simulink model "SIL_OlfatiSaber"  (R2021b)
settings: Solver=FixedStepDiscrete  StartTime=0  StopTime=T  FixedStep=0.01  RelTol=1e-3  EnableMultiTasking=on
model workspace (MAT data in the model file):
  SL_ROS_VariableLengthArrays_MaxSizes : object (value not decoded)
values from neighbouring files (symbols this model uses):
  airspeed_ref = 42    [start_swarm.m]
  altitude_ref = 300    [start_swarm.m]
  N_Waypoints = size(Waypoints,1)    [start_swarm.m]
  radius_waypoint = 200    [start_swarm.m]
  Waypoints = [1200 -1000 ... (first row only)    [start_swarm.m]
undefined symbols (not defined in the file or in its folder): DiscIntNeverNeededParam, Elevators, p_swarm, Propeller, RightAileron, RightFlap, Rudder
libraries: robotlib x36, slpidlib x15, eeGeneralControl x5, simulink x5
(part 4 of 5)

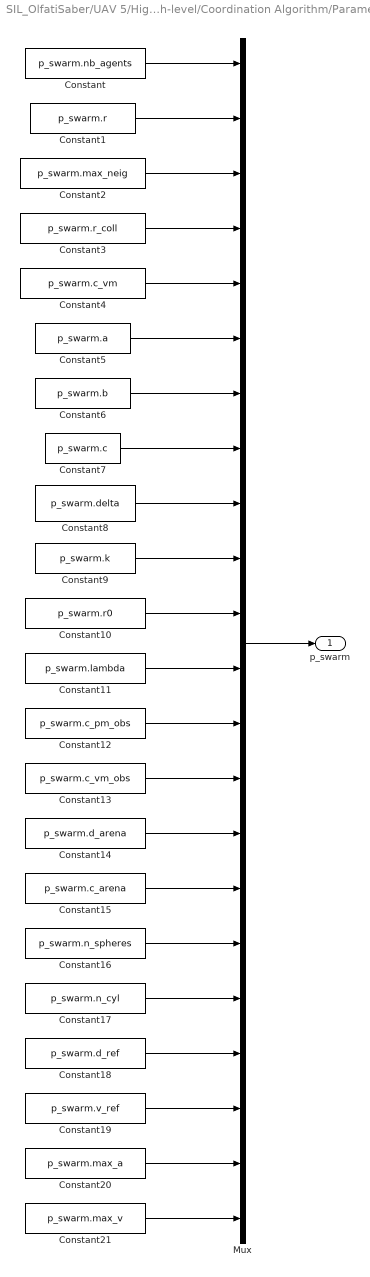
== system SIL_OlfatiSaber/UAV 5/High-level/Coordination Algorithm/Parameters ==
  Constant : Constant  Value=p_swarm.nb_agents
  Constant1 : Constant  Value=p_swarm.r
  Constant10 : Constant  Value=p_swarm.r0
  Constant11 : Constant  Value=p_swarm.lambda
  Constant12 : Constant  Value=p_swarm.c_pm_obs
  Constant13 : Constant  Value=p_swarm.c_vm_obs
  Constant14 : Constant  Value=p_swarm.d_arena
  Constant15 : Constant  Value=p_swarm.c_arena
  Constant16 : Constant  Value=p_swarm.n_spheres
  Constant17 : Constant  Value=p_swarm.n_cyl
  Constant18 : Constant  Value=p_swarm.d_ref
  Constant19 : Constant  Value=p_swarm.v_ref
  Constant2 : Constant  Value=p_swarm.max_neig
  Constant20 : Constant  Value=p_swarm.max_a
  Constant21 : Constant  Value=p_swarm.max_v
  Constant3 : Constant  Value=p_swarm.r_coll
  Constant4 : Constant  Value=p_swarm.c_vm
  Constant5 : Constant  Value=p_swarm.a
  Constant6 : Constant  Value=p_swarm.b
  Constant7 : Constant  Value=p_swarm.c
  Constant8 : Constant  Value=p_swarm.delta
  Constant9 : Constant  Value=p_swarm.k
  Mux : Mux  Inputs=22
  p_swarm : Outport
  wires:
  Mux/1 -> p_swarm/1
  Constant21/1 -> Mux/22
  Constant20/1 -> Mux/21
  Constant19/1 -> Mux/20
  Constant18/1 -> Mux/19
  Constant17/1 -> Mux/18
  Constant16/1 -> Mux/17
  Constant15/1 -> Mux/16
  Constant14/1 -> Mux/15
  Constant13/1 -> Mux/14
  Constant12/1 -> Mux/13
  Constant11/1 -> Mux/12
  Constant10/1 -> Mux/11
  Constant9/1 -> Mux/10
  Constant8/1 -> Mux/9
  Constant7/1 -> Mux/8
  Constant6/1 -> Mux/7
  Constant5/1 -> Mux/6
  Constant4/1 -> Mux/5
  Constant3/1 -> Mux/4
  Constant2/1 -> Mux/3
  Constant1/1 -> Mux/2
  Constant/1 -> Mux/1

== system SIL_OlfatiSaber/UAV 5/Low-level/Autopilot/Altitude Control ==
  Altitude Ref : Inport
  Altitude : Inport  Port=2
  Constant : Constant
  Constant1 : Constant  Value=0.00
  Constant2 : Constant  Value=0.0162
  Constant3 : Constant  Value=10
  Discrete PID : slpidlib/PID Controller  Controller=PID  Form=Parallel  TimeDomain=Discrete-time  UseExternalTs=off  SampleTime=-1  IntegratorMethod=Forward Euler  FilterMethod=Forward Euler  ControllerParametersSource=external  P=1  I=1  D=0  UseFilter=on  N=100  TunerSelectOption=Transfer Function Based (PID Tuner App)  InitialConditionSource=internal  InitialConditionForIntegrator=0  InitialConditionForFilter=0  DifferentiatorICPrevScaledInput=0  ExternalReset=none  TrackingMode=off  Kt=1  LimitOutput=off  SatLimitsSource=internal  UpperSaturationLimit=inf  LowerSaturationLimit=-inf  LinearizeAsGain=on  AntiWindupMode=none  Kb=1  POutMin=[]  POutMax=[]  IOutMin=[]  IOutMax=[]  DOutMin=[]  DOutMax=[]  NOutMin=[]  NOutMax=[]  SumOutMin=[]  SumOutMax=[]  SaturationOutMin=[]  SaturationOutMax=[]  PParamMin=[]  PParamMax=[]  IParamMin=[]  IParamMax=[]  DParamMin=[]  DParamMax=[]  NParamMin=[]  NParamMax=[]  KbParamMin=[]  KbParamMax=[]  KtParamMin=[]  KtParamMax=[]  KbOutMin=[]  KbOutMax=[]  KtOutMin=[]  KtOutMax=[]  IntegratorOutMin=[]  IntegratorOutMax=[]  FilterOutMin=[]  FilterOutMax=[]  SumI1OutMin=[]  SumI1OutMax=[]  SumI2OutMin=[]  SumI2OutMax=[]  SumI3OutMin=[]  SumI3OutMax=[]  SumI4OutMin=[]  SumI4OutMax=[]  SumDOutMin=[]  SumDOutMax=[]  DifferentiatorOutMin=[]  DifferentiatorOutMax=[]  FilterDiffOutCoefMin=[]  FilterDiffOutCoefMax=[]  ReciprocalOutMin=[]  ReciprocalOutMax=[]  SumDenOutMin=[]  SumDenOutMax=[]  SumNumOutMin=[]  SumNumOutMax=[]  DivideOutMin=[]  DivideOutMax=[]  UdiffTsProdOutMin=[]  UdiffTsProdOutMax=[]  NTsProdOutMin=[]  NTsProdOutMax=[]  UintegralTsProdOutMin=[]  UintegralTsProdOutMax=[]  UngainTsProdOutMin=[]  UngainTsProdOutMax=[]  IntegratorContinuousStateAttributes=''  IntegratorStateMustResolveToSignalObject=off  IntegratorRTWStateStorageClass=Auto  FilterContinuousStateAttributes=''  FilterStateMustResolveToSignalObject=off  FilterRTWStateStorageClass=Auto  ParallelPVariant=ExternalParameters  IdealPVariant=Disabled  IVariant=ExternalParameters  DVariant=ExternalParameters  IntegratorVariant=Discrete  SatVariant=Disabled  AWVariant=Passthrough  PCopyVariant=Disabled  TRVariant=Disabled  FdbkBlocksVariant=Forward  IdealPFdbkVariant=Disabled  SatFdbkVariant=Disabled  DerivativeFilterVariant=ForwardEulerFilter  NVariant=ExternalParameters  NCopyVariant=Disabled  FilterICVariant=InternalICsFilter  IntegratorICVariant=InternalICs  ExternalResetVariant=Disabled  TRSumVariant=Passthrough  SumFdbkVariant=Disabled  SumVariant=Sum_PID  TsampFilterVariant=InternalTs  TsampNgainVariant=Passthrough  TsampIntegralVariant=Passthrough  ExternalSaturationOutDataTypeStr=Inherit: Same as second input
  Gain : Gain  Gain=0.1
  Saturation : Saturate  UpperLimit=0.78  LowerLimit=-0.78
  Sum : Sum  Inputs=|+-
  Pitch_ref : Outport
  altitude_error : Outport  Port=2
  wires:
  Saturation/1 -> Pitch_ref/1
  Altitude Ref/1 -> Sum/1
  Altitude/1 -> Sum/2
  Sum/1 -> altitude_error/1, Gain/1
  Constant/1 -> Discrete PID/2
  Constant1/1 -> Discrete PID/3
  Constant2/1 -> Discrete PID/4
  Constant3/1 -> Discrete PID/5
  Discrete PID/1 -> Saturation/1
  Gain/1 -> Discrete PID/1

== system SIL_OlfatiSaber/UAV 5/Low-level/Autopilot/Attitude Control ==
  Pitch Ref : Inport
  Roll_ref : Inport  Port=2
  Euler angles : Inport  Port=3
  Bus Selector1 : BusSelector  OutputSignals=Pitch,Yaw,Roll
  Sum1 : Sum  Inputs=|+-
  Sum3 : Sum  Inputs=+-|
  Terminator : Terminator
  pitch_error : Outport
  roll_error : Outport  Port=2
  wires:
  Euler angles/1 -> Bus Selector1/1
  Sum1/1 -> roll_error/1
  Sum3/1 -> pitch_error/1
  Roll_ref/1 -> Sum1/1
  Bus Selector1/1 -> Sum3/2  "<Pitch>"
  Pitch Ref/1 -> Sum3/1
  Bus Selector1/3 -> Sum1/2  "<Roll>"
  Bus Selector1/2 -> Terminator/1  "<Yaw>"

== system SIL_OlfatiSaber/UAV 5/Low-level/Autopilot/Takeoff ==
  Elevator Command : Inport
  Ailerons Command : Inport  Port=2
  Propeller Command : Inport  Port=3
  Altitude : Inport  Port=4
  Constant1 : Constant  Value=0.0436332
  Constant2 : Constant  Value=0.017
  Constant3 : Constant  Value=0.8
  Constant4 : Constant  Value=0
  Constant5 : Constant  Value=-0.035
  GreaterThanOrEqual : RelationalOperator  OutDataTypeStr=boolean  RndMeth=Simplest
  Switch{1..4} (4 alike) : Switch  Criteria=u2 ~= 0
  altitude takeoff : Constant  Value=5
  profundor : Outport
  aileron : Outport  Port=2
  throtlle : Outport  Port=3
  rudder : Outport  Port=4
  wires:
  Elevator Command/1 -> Switch3/1
  Switch3/1 -> profundor/1
  Ailerons Command/1 -> Switch1/1
  Switch1/1 -> aileron/1
  Switch2/1 -> throtlle/1
  Propeller Command/1 -> Switch2/1
  Constant1/1 -> Switch3/3
  Constant2/1 -> Switch1/3
  Constant3/1 -> Switch2/3
  altitude takeoff/1 -> GreaterThanOrEqual/2
  Altitude/1 -> GreaterThanOrEqual/1
  GreaterThanOrEqual/1 -> Switch4/2, Switch3/2, Switch1/2, Switch2/2
  Constant4/1 -> Switch4/1
  Constant5/1 -> Switch4/3
  Switch4/1 -> rudder/1

== system SIL_OlfatiSaber/UAV 5/Low-level/Autopilot/Velocity Control ==
  Velocity Ref : Inport
  Velocity : Inport  Port=2
  Constant : Constant
  Constant1 : Constant  Value=0.00
  Constant2 : Constant  Value=0.009
  Constant3 : Constant  Value=10
  Discrete PID : slpidlib/PID Controller  Controller=PID  Form=Parallel  TimeDomain=Discrete-time  UseExternalTs=off  SampleTime=-1  IntegratorMethod=Forward Euler  FilterMethod=Forward Euler  ControllerParametersSource=external  P=1  I=1  D=0  UseFilter=on  N=100  TunerSelectOption=Transfer Function Based (PID Tuner App)  InitialConditionSource=internal  InitialConditionForIntegrator=0  InitialConditionForFilter=0  DifferentiatorICPrevScaledInput=0  ExternalReset=none  TrackingMode=off  Kt=1  LimitOutput=off  SatLimitsSource=internal  UpperSaturationLimit=inf  LowerSaturationLimit=-inf  LinearizeAsGain=on  AntiWindupMode=none  Kb=1  POutMin=[]  POutMax=[]  IOutMin=[]  IOutMax=[]  DOutMin=[]  DOutMax=[]  NOutMin=[]  NOutMax=[]  SumOutMin=[]  SumOutMax=[]  SaturationOutMin=[]  SaturationOutMax=[]  PParamMin=[]  PParamMax=[]  IParamMin=[]  IParamMax=[]  DParamMin=[]  DParamMax=[]  NParamMin=[]  NParamMax=[]  KbParamMin=[]  KbParamMax=[]  KtParamMin=[]  KtParamMax=[]  KbOutMin=[]  KbOutMax=[]  KtOutMin=[]  KtOutMax=[]  IntegratorOutMin=[]  IntegratorOutMax=[]  FilterOutMin=[]  FilterOutMax=[]  SumI1OutMin=[]  SumI1OutMax=[]  SumI2OutMin=[]  SumI2OutMax=[]  SumI3OutMin=[]  SumI3OutMax=[]  SumI4OutMin=[]  SumI4OutMax=[]  SumDOutMin=[]  SumDOutMax=[]  DifferentiatorOutMin=[]  DifferentiatorOutMax=[]  FilterDiffOutCoefMin=[]  FilterDiffOutCoefMax=[]  ReciprocalOutMin=[]  ReciprocalOutMax=[]  SumDenOutMin=[]  SumDenOutMax=[]  SumNumOutMin=[]  SumNumOutMax=[]  DivideOutMin=[]  DivideOutMax=[]  UdiffTsProdOutMin=[]  UdiffTsProdOutMax=[]  NTsProdOutMin=[]  NTsProdOutMax=[]  UintegralTsProdOutMin=[]  UintegralTsProdOutMax=[]  UngainTsProdOutMin=[]  UngainTsProdOutMax=[]  IntegratorContinuousStateAttributes=''  IntegratorStateMustResolveToSignalObject=off  IntegratorRTWStateStorageClass=Auto  FilterContinuousStateAttributes=''  FilterStateMustResolveToSignalObject=off  FilterRTWStateStorageClass=Auto  ParallelPVariant=ExternalParameters  IdealPVariant=Disabled  IVariant=ExternalParameters  DVariant=ExternalParameters  IntegratorVariant=Discrete  SatVariant=Disabled  AWVariant=Passthrough  PCopyVariant=Disabled  TRVariant=Disabled  FdbkBlocksVariant=Forward  IdealPFdbkVariant=Disabled  SatFdbkVariant=Disabled  DerivativeFilterVariant=ForwardEulerFilter  NVariant=ExternalParameters  NCopyVariant=Disabled  FilterICVariant=InternalICsFilter  IntegratorICVariant=InternalICs  ExternalResetVariant=Disabled  TRSumVariant=Passthrough  SumFdbkVariant=Disabled  SumVariant=Sum_PID  TsampFilterVariant=InternalTs  TsampNgainVariant=Passthrough  TsampIntegralVariant=Passthrough  ExternalSaturationOutDataTypeStr=Inherit: Same as second input
  K_prop : Gain  Gain=0.1
  Sum1 : Sum  Inputs=|++
  Sum7 : Sum  Inputs=|+-
  propeller_ref : Constant  Value=0.64
  propeller_cmd : Outport
  velocity_error : Outport  Port=2
  wires:
  Velocity/1 -> Sum7/2
  Velocity Ref/1 -> Sum7/1
  Sum7/1 -> velocity_error/1, K_prop/1
  Sum1/1 -> propeller_cmd/1
  propeller_ref/1 -> Sum1/2
  Constant3/1 -> Discrete PID/5
  Constant/1 -> Discrete PID/2
  Discrete PID/1 -> Sum1/1
  Constant1/1 -> Discrete PID/3
  K_prop/1 -> Discrete PID/1
  Constant2/1 -> Discrete PID/4

== matlab function SIL_OlfatiSaber/UAV 1/High-level/Waypoint Generator/Velocity Direction ==
  data: pos input; wp input; u_ref output
function u_ref = velocity_direction(pos, wp)
    pos_mean_rel = wp - pos;
    
    r = sqrt( sum( pos_mean_rel.^2 ) );
    x = pos_mean_rel(1);
    y = pos_mean_rel(2);
    %z = pos_mean_rel(3)/r;
    
    orientation = atan2(y,x);
    u_ref = [cos(orientation); sin(orientation); 0];

end

== matlab function SIL_OlfatiSaber/UAV 2/High-level/Network/Status Network ==
  data: N_Agents input; Wifi_Scan input; SignalDbms output
% this function is a union of data of uav i and your neighbors
function SignalDbms = Wifi_Signal(N_Agents, Wifi_Scan)
    SignalDbms = zeros(1, 5);
    Ssids = zeros(1, 5);
    Frequencys = zeros(1, 5);
    
    for i=1:N_Agents
        SignalDbms(i) = Wifi_Scan.Signals(i).SignalDbm;
        %Ssids(i) = Wifi_Scan.Signals(i).Ssid;
        %Frequencys(i) = Wifi_Scan.Signals(i).Frequency;
    end
end

== matlab function SIL_OlfatiSaber/UAV 2/High-level/Waypoint Generator/Velocity Direction ==
  data: pos input; wp input; u_ref output
function u_ref = velocity_direction(pos, wp)
    pos_mean_rel = wp - pos;
    
    r = sqrt( sum( pos_mean_rel.^2 ) );
    x = pos_mean_rel(1);
    y = pos_mean_rel(2);
    %z = pos_mean_rel(3)/r;
    
    orientation = atan2(y,x);
    u_ref = [cos(orientation); sin(orientation); 0];

end

== matlab function SIL_OlfatiSaber/UAV 2/High-level/Waypoint Generator/Waypoint Algorithm ==
  data: Xi input; R input; p_swarm_r input; Waypoints input; N_Waypoints input; wp output; Current_Waypoint output; Current_Waypoint input
function [wp, Current_Waypoint] = Next_Waypoint(Xi, R, p_swarm_r, Waypoints, N_Waypoints, Current_Waypoint)

    X_ref = Waypoints(Current_Waypoint + 1, 1);
    Y_ref = Waypoints(Current_Waypoint + 1, 2);
    wp = [X_ref; Y_ref; 0];

    if ( is_visited(Xi, R, p_swarm_r, X_ref, Y_ref)  )
        Current_Waypoint = mod(Current_Waypoint + 1, N_Waypoints);
    else
        Current_Waypoint = mod(Current_Waypoint, N_Waypoints);
    end

end

function visited = is_visited(Xi, R, p_swarm_r, wp1_X,wp1_Y)
    visited = 0;
    N = size(Xi,2);
    
    for i=1:N
        % if the aircraft inter the communication range and acces the
        % waypoitn area
        if( sqrt( (Xi(1, 1) - Xi(1, i) )^2 +(Xi(2, 1) - Xi(2, i))^2) < p_swarm_r && sqrt( (wp1_X - Xi(1, i) )^2 +(wp1_Y - Xi(2, i))^2) < R )
            visited = 1;
            return
        end
    end
    
end

== matlab function SIL_OlfatiSaber/UAV 2/Low-level/ROS Settings/Wi-Fi frame to Matrix ==
  data: nb_agents input; pos_i input; pos output; pqj input
% this function is a union of data of uav i and your neighbors
function pos = uavs_data(nb_agents, pos_i, pqj)
    %% Create Matrix pj and qj neighbors
    nb_agents = 5;
    
    pos = zeros(3, nb_agents);  % 
    %vel = zeros(3, nb_agents);  % 
    
    % position of agent i
    pos(:,1) = pos_i; % Posição
    %vel(:,1) = vel_i; % Velocidade
    
    % neighbors of i
    for j=1:nb_agents-1
         %id_j = pqj(j).Id;
         pos(:,j+1) = [pqj(j).X; pqj(j).Y; pqj(j).Z]; % Posição
         %vel(:,j+1) = [pqj(j).VelocityX; pqj(j).VelocityY; pqj(j).VelocityZ]; % Velocidade
    end

end

== matlab function SIL_OlfatiSaber/UAV 3/High-level/Coordination Algorithm/Olfati-Saber Algorithm ==
  data: p_swarm_par input; pos input; vel input; u_ref input; dt input; r_agent input; vel_command output
function vel_command = compute_vel_olfati_saber(p_swarm_par, pos, vel, u_ref, dt, r_agent)
    
    %% swarm parameters
    % variables to be set
    p_swarm.is_active_migration = 1;
    p_swarm.is_active_arena = 0;
    p_swarm.is_active_spheres = 0;
    p_swarm.is_active_cyl = 0;
    
    % number of agents
    nb_agents = 5;
    
    % max radius of influence - metric distance
    p_swarm.r = p_swarm_par(2);
    
    % max number of neighbors - Topological distance
    p_swarm.max_neig = p_swarm_par(3);
    
    % radius of collision
    p_swarm.r_coll = p_swarm_par(4);
    
    % % Olfati-Saber parameters
    % coefficients for velocity matching
    p_swarm.c_vm = p_swarm_par(5);
    p_swarm.a = p_swarm_par(6);
    p_swarm.b = p_swarm_par(7);
    p_swarm.c = p_swarm_par(8); %(p_swarm.b-p_swarm.a)/(2*sqrt(p_swarm.a*p_swarm.b));
    p_swarm.delta = p_swarm_par(9);
    p_swarm.k = p_swarm_par(10);
    
    % obstacle parameters
    p_swarm.r0 = p_swarm_par(11);
    p_swarm.lambda = p_swarm_par(12); % (0,1]
    p_swarm.c_pm_obs = p_swarm_par(13);
    p_swarm.c_vm_obs = p_swarm_par(14); %p_swarm.c_vm;
    
    % wall parameters
    p_swarm.d_arena = p_swarm_par(15);
    p_swarm.c_arena = p_swarm_par(16);
    p_swarm.n_spheres = p_swarm_par(17);
    p_swarm.n_cyl = p_swarm_par(18);
    p_swarm.spheres = [-70 70 0; 50 50 200; 5 5 5; 50 50 50];
    p_swarm.x_arena = [-100   100; -100   100; -100   100];
    p_swarm.cylinders = [];
    
    % % Reference values

    % Inter-agent distance
    p_swarm.d_ref = p_swarm_par(19);
    
    % Velocity direction
    p_swarm.u_ref = u_ref;

    % Speed
    p_swarm.v_ref = p_swarm_par(20);
    
    % Velocity and acceleration bounds for the agents
    p_swarm.max_a = p_swarm_par(21);
    p_swarm.max_v = p_swarm_par(22);

    %% Initialize variables
    
    M = zeros(1, nb_agents);    % Neighborhood matrix
    D = zeros(1, nb_agents);    % Distance matrix
    acc_pm = zeros(3, 1);       % Position matching acceleration
    acc_vm = zeros(3, 1);       % Velocity matching acceleration
    acc_wall = zeros(3, 1);     % Arena repulsion acceleration
    acc_obs = zeros(3, 1);      % Obstacle repulsion acceleration
    acc_command = zeros(3, 1);  % Calculate the commanded acceleration
    vel_command = zeros(3, 1);  % Calculate the commanded velocity

    nb_agent_collisions = 0;    % Nb of collisions among agents
    nb_obs_collisions = 0;      % Nb of collisions against obstacles
    min_dist_obs = 20;          % Init minimum distance to obstacles

    %% Compute useful functions

    % Weight function for computing the motion planning acceleration
    psi = @(z) ((p_swarm.a + p_swarm.b) * (sqrt(1 + (z - p_swarm.d_ref + p_swarm.c)^2) - sqrt(1 + p_swarm.c^2)) + ...
        (p_swarm.a - p_swarm.b) * (z - p_swarm.d_ref)) / 2;
    psi_der = @(z) (p_swarm.a + p_swarm.b) / 2 * (z - p_swarm.d_ref + p_swarm.c) ./ sqrt(1 + (z - p_swarm.d_ref + p_swarm.c)^2) + ...
        (p_swarm.a - p_swarm.b) / 2;

    % Generalization of adjacency coefficients for computing the motion planning acceleration
    rho = @rho_f;
    rho_der = @rho_der_f;

    % Force defining the attraction/repulsion as function of the distance
    phi = @(z) 1 / p_swarm.r * rho_der(z, p_swarm.delta, p_swarm.r, p_swarm.k) * psi(z) + ...
        rho(z, p_swarm.delta, p_swarm.r, p_swarm.k) * psi_der(z);
   
%% Compute velocity commands for every agent
    
    for agent = 1:1
        
        
        %% Find neighbors
        
        % Compute agent-agent distance matrix
        % p_rel = pos - pos(:, agent);
        p_rel = zeros(3, nb_agents);
        for k = 1:nb_agents
            p_rel(:, k) = pos(:, k) - pos(:, agent);
        end
        
        dist = sqrt(sum((p_rel.^2), 1));
        D(agent, :) = dist;

        % Define neighbors list
        neig_lis = (1:nb_agents)';
        neig_lis = neig_lis(dist ~= 0);

        % Count collisions
        nb_agent_collisions = nb_agent_collisions + sum(dist < 2 * r_agent) - 1;

        % Number of neighbours
        nb_neig = nb_agents - 1;

        % Constraint on neighborhood given by the euclidean distance
        if isfield(p_swarm, 'r')
            neig_lis = neig_lis(dist(neig_lis) < p_swarm.r);
            nb_neig = length(neig_lis);
        end

        % Constraint on neighborhood given by the topological distance
        if isfield(p_swarm, 'max_neig')

            if nb_neig > p_swarm.max_neig
                [~, idx] = sort(dist(neig_lis));
                neig_lis = neig_lis(idx(1:p_swarm.max_neig));
                nb_neig = p_swarm.max_neig;
            end

        end

        % Adjacency matrix (asymmetric in case of limited fov)
        M(agent, neig_lis) = 1;

        
        %% Compute different contributions
        if nb_neig ~= 0
            % vel_rel = vel - vel(:, agent);
            vel_rel = zeros(3, nb_agents);
            for k = 1:nb_agents
                vel_rel(:, k) = vel(:, k) - vel(:, agent);
            end
            % v_rel_norm  = sqrt(sum((v_rel.^2),1));

            % Compute pos unit vector between two agents
            %pos_rel_u = p_rel ./ dist;
            pos_rel_u = zeros(3, nb_agents); 
            for k = 1:nb_agents
                if(k ~= agent)
                    pos_rel_u(:, k) = p_rel(:, k) ./ dist(k);
                end
            end
            
            for agent2 = 1:nb_agents
                % Position matching
                acc_pm(:, agent) = acc_pm(:, agent) + phi(dist(agent2)) * pos_rel_u(:, agent2);

                % Velocity matching
                if ~p_swarm.is_active_migration
                    acc_vm(:, agent) = acc_vm(:, agent) + p_swarm.c_vm * vel_rel(agent2);
                end
            end
        end

        % Add migration effect on accelerations
        if p_swarm.is_active_migration
            acc_vm(:, agent) = p_swarm.c_vm * (p_swarm.u_ref * p_swarm.v_ref - vel(:, agent));
        end
        
        
        %% Wall and obstacle avoidance

        % Add arena repulsion effect on accelerations
        if p_swarm.is_active_arena
            acc_wall(:, agent) = repulsion_cubic_arena(pos(:, agent), p_swarm.x_arena, p_swarm.d_arena, p_swarm.c_arena);
        end

        % Spheric obstacles effect
        if p_swarm.is_active_spheres

            for obs = 1:p_swarm.n_spheres
                % Get obstacle center and radius
                c_obs = p_swarm.spheres(1:3, obs);
                r_obs = p_swarm.spheres(4, obs);

                pos_agent = pos(:, agent);
                vel_agent = vel(:, agent);

                % Compute distance agent(a)-obstacle(b)
                dist_ab = sqrt(sum((pos(:, agent) - c_obs).^2)) - r_obs;
                nb_obs_collisions = nb_obs_collisions + sum(dist_ab < r_agent);

                if dist_ab < min_dist_obs
                    min_dist_obs = dist_ab;
                end

                if (dist_ab < p_swarm.r0)
                    % Parameter s in [0,1]
                    s = r_obs / (r_obs + dist_ab);
                    pos_obs = s * pos_agent + (1 - s) * c_obs;

                    % Derivative of s
                    s_dot = r_obs * (vel_agent' * (pos_obs - pos_agent) / dist_ab) / (r_obs + dist_ab)^2;
                    vel_obs = s * vel_agent - r_obs * (s_dot / s) * (pos_obs - pos_agent) / dist_ab;
                    pos_gamma = c_obs + p_swarm.lambda * p_swarm.u_ref;
                    d_ag = norm(pos_gamma - pos(:, agent));

                    % Acceleration effect
                    acc_obs(:, agent) = acc_obs(:, agent) + ...
                        +p_swarm.c_pm_obs * rho(dist_ab / p_swarm.r0, p_swarm.delta, p_swarm.r, p_swarm.k) * ...
                        (phi(dist_ab - p_swarm.d_ref) * (pos_obs - pos_agent) / dist_ab + ...
                        phi(d_ag - p_swarm.d_ref) * (pos_gamma - pos_agent) / (norm(pos_gamma - pos_agent))) + ...
                        p_swarm.c_vm_obs * (vel_obs - vel_agent);
                end
            end
        end

        % Cylindric obstacle effect
        if p_swarm.is_active_cyl

            for obs = 1:p_swarm.n_cyl
                % Get obstacle center and radius
                c_obs = p_swarm.cylinders(1:2, obs);
                r_obs = p_swarm.cylinders(3, obs);

                pos_agent = pos(1:2, agent);
                vel_agent = vel(1:2, agent);

                % Compute distance agent(a)-obstacle(b)
                dist_ab = sqrt(sum((pos(1:2, agent) - c_obs).^2)) - r_obs;
                nb_obs_collisions = nb_obs_collisions + sum(dist_ab < r_agent);

                if dist_ab < min_dist_obs
                    min_dist_obs = dist_ab;
                end

                % Compute interaction effect
                if (dist_ab < p_swarm.r0)
                    % Parameter s in [0,1]
                    s = r_obs / (r_obs + dist_ab);
                    pos_obs = s * pos_agent + (1 - s) * c_obs;

                    % Derivative of s
                    s_dot = r_obs * (vel_agent' * (pos_obs - pos_agent) / dist_ab) / (r_obs + dist_ab)^2;
                    vel_obs = s * vel_agent - r_obs * (s_dot / s) * (pos_obs - pos_agent) / dist_ab;
                    pos_gamma = c_obs + p_swarm.lambda * p_swarm.u_ref(1:2);
                    d_ag = norm(pos_gamma - pos(1:2, agent));

                    % Acceleration effect of the spheric obstacles
                    acc_obs(1:2, agent) = acc_obs(1:2, agent) + ...
                        +p_swarm.c_pm_obs * rho(dist_ab / p_swarm.r0, p_swarm.delta, p_swarm.r, p_swarm.k) * ...
                        (phi(dist_ab - p_swarm.d_ref) * (pos_obs - pos_agent) / dist_ab + ...
                        phi(d_ag - p_swarm.d_ref) * (pos_gamma - pos_agent) / (norm(pos_gamma - pos_agent))) + ...
                        p_swarm.c_vm_obs * (vel_obs - vel_agent);
                end

            end

        end
        
        %% Sum contributions
        acc_command(:, agent) = acc_pm(:, agent) + acc_vm(:, agent) + acc_wall(:, agent) + acc_obs(:, agent); 
        
        % Integrate acceleration to get velocity
        vel_command(:, agent) = vel(:, agent) + acc_command(:, agent) * dt;
        
    end
    
    %% Compute collisions and bound velocities and accelerations
    
    % Add random effect on velocities
    if isfield(p_swarm, 'c_r')
        vel_command = vel_command + p_swarm.c_r * randn(3, nb_agents);
    end

    % Bound velocities
    if isempty(p_swarm.max_v)
        v_norm = sqrt(sum((vel_command.^2), 1));
        idx_to_bound = (v_norm > p_swarm.max_v);

        if sum(idx_to_bound) > 0
            vel_command(:, idx_to_bound) = p_swarm.max_v * ...
                vel_command(:, idx_to_bound) ./ repmat(v_norm(idx_to_bound), 3, 1);
        end
    end
    if isempty(p_swarm.max_a)
        accel_cmd = (vel_command-vel)./dt;
        accel_cmd_norm = sqrt(sum(accel_cmd.^2, 1));
        idx_to_bound = ( accel_cmd_norm > p_swarm.max_a | accel_cmd_norm < - p_swarm.max_a);
        if sum(idx_to_bound) > 0
            vel_command(:, idx_to_bound) = vel(:, idx_to_bound) + ...
                dt*p_swarm.max_a * accel_cmd(:, idx_to_bound) ./ ...
                repmat(accel_cmd_norm(idx_to_bound), 3, 1);
        end
    end

end

%%%%%%%%%%%%%%%%%%%%%%%%%%%%%%%%%%%%%%%%%%%%%%%%%%
% RHO - It is the function defining the adjacency coefficients
%
%%%%%%%%%%%%%%%%%%%%%%%%%%%%%%%%%%%%%%%%%%%%%%%%%%

function y = rho_f(z, delta, r, k)

    if z < delta * r
        y = 1;
        return;
    elseif z < r
        y = (1/2^k) * (1 + cos(pi * (z / r - delta) ./ (1 - delta)))^k;
        return;
    else
        y = 0;
    end

end

%%%%%%%%%%%%%%%%%%%%%%%%%%%%%%%%%%%%%%%%%%%%%%%%%%
% Derivative of rho
%
%%%%%%%%%%%%%%%%%%%%%%%%%%%%%%%%%%%%%%%%%%%%%%%%%%

function y = rho_der_f(z, delta, r, k)

    if z < delta * r
        y = 0;
        return;
    elseif z < r
        arg = pi * (z / r - delta) ./ (1 - delta);
        y = -pi / (1 - delta) * k / (2^k) * (1 + cos(arg))^(k - 1) * (sin(arg));
        return;
    else
        y = 0;
    end

end

%%%%%%%%%%%%%%%%%%%%%%%%%%%%%%%%%%%%%%%%%%%%%%%%%%
% Repulsion from cubic arena
%
%%%%%%%%%%%%%%%%%%%%%%%%%%%%%%%%%%%%%%%%%%%%%%%%%%

function a_arena = repulsion_cubic_arena(pos_drone, pos_walls, wall_width, const_rep)

    a_arena = zeros(3, 1);

    for axis = 1:3
        x_drone = pos_drone(axis);
        % Repulsion from left wall
        x_arena = pos_walls(axis, 1);

        if x_drone < x_arena
            a_arena(axis) = a_arena(axis) + const_rep;
        elseif x_drone > x_arena && x_drone < x_arena + wall_width
            a_arena(axis) = a_arena(axis) + const_rep * 0.5 * (sin((pi / wall_width) * (x_drone + x_arena) + pi / 2) + 1);
        end

        % Repulsion from right wall
        x_arena = pos_walls(axis, 2);

        if x_drone > x_arena - wall_width && x_drone < x_arena
            a_arena(axis) = a_arena(axis) - const_rep * 0.5 * (sin((pi / wall_width) * (x_drone - x_arena - wall_width) - pi / 2) + 1);
        elseif x_drone > x_arena
            a_arena(axis) = a_arena(axis) - const_rep;
        end

    end

end

== matlab function SIL_OlfatiSaber/UAV 3/High-level/Network/Status Network ==
  data: N_Agents input; Wifi_Scan input; SignalDbms output
% this function is a union of data of uav i and your neighbors
function SignalDbms = Wifi_Signal(N_Agents, Wifi_Scan)
    SignalDbms = zeros(1, 5);
    Ssids = zeros(1, 5);
    Frequencys = zeros(1, 5);
    
    for i=1:N_Agents
        SignalDbms(i) = Wifi_Scan.Signals(i).SignalDbm;
        %Ssids(i) = Wifi_Scan.Signals(i).Ssid;
        %Frequencys(i) = Wifi_Scan.Signals(i).Frequency;
    end
end

== matlab function SIL_OlfatiSaber/UAV 3/High-level/Waypoint Generator/Velocity Direction ==
  data: pos input; wp input; u_ref output
function u_ref = velocity_direction(pos, wp)
    pos_mean_rel = wp - pos;
    
    r = sqrt( sum( pos_mean_rel.^2 ) );
    x = pos_mean_rel(1);
    y = pos_mean_rel(2);
    %z = pos_mean_rel(3)/r;
    
    orientation = atan2(y,x);
    u_ref = [cos(orientation); sin(orientation); 0];

end

== matlab function SIL_OlfatiSaber/UAV 3/High-level/Waypoint Generator/Waypoint Algorithm ==
  data: Xi input; R input; p_swarm_r input; Waypoints input; N_Waypoints input; wp output; Current_Waypoint output; Current_Waypoint input
function [wp, Current_Waypoint] = Next_Waypoint(Xi, R, p_swarm_r, Waypoints, N_Waypoints, Current_Waypoint)

    X_ref = Waypoints(Current_Waypoint + 1, 1);
    Y_ref = Waypoints(Current_Waypoint + 1, 2);
    wp = [X_ref; Y_ref; 0];

    if ( is_visited(Xi, R, p_swarm_r, X_ref, Y_ref)  )
        Current_Waypoint = mod(Current_Waypoint + 1, N_Waypoints);
    else
        Current_Waypoint = mod(Current_Waypoint, N_Waypoints);
    end

end

function visited = is_visited(Xi, R, p_swarm_r, wp1_X,wp1_Y)
    visited = 0;
    N = size(Xi,2);
    
    for i=1:N
        % if the aircraft inter the communication range and acces the
        % waypoitn area
        if( sqrt( (Xi(1, 1) - Xi(1, i) )^2 +(Xi(2, 1) - Xi(2, i))^2) < p_swarm_r && sqrt( (wp1_X - Xi(1, i) )^2 +(wp1_Y - Xi(2, i))^2) < R )
            visited = 1;
            return
        end
    end
    
end

== matlab function SIL_OlfatiSaber/UAV 3/Low-level/ROS Settings/Wi-Fi frame to Matrix ==
  data: nb_agents input; pos_i input; pos output; pqj input
% this function is a union of data of uav i and your neighbors
function pos = uavs_data(nb_agents, pos_i, pqj)
    %% Create Matrix pj and qj neighbors
    nb_agents = 5;
    
    pos = zeros(3, nb_agents);  % 
    %vel = zeros(3, nb_agents);  % 
    
    % position of agent i
    pos(:,1) = pos_i; % Posição
    %vel(:,1) = vel_i; % Velocidade
    
    % neighbors of i
    for j=1:nb_agents-1
         %id_j = pqj(j).Id;
         pos(:,j+1) = [pqj(j).X; pqj(j).Y; pqj(j).Z]; % Posição
         %vel(:,j+1) = [pqj(j).VelocityX; pqj(j).VelocityY; pqj(j).VelocityZ]; % Velocidade
    end

end

== matlab function SIL_OlfatiSaber/Save Data/Positions Plot ==
  data: Positions input
function plotFormation(Positions)
persistent p;

Pos1 = reshape(Positions,3,[]);

if isempty(p)
    %hold on
    p = plot(Pos1(1,:), Pos1(2,:), 'ro', 'MarkerSize',15);
    %w = plot(Position(1), Position(2), 'b*');
    %hold off
    %set(gca,'XLim', [-3000 3000], 'YLim', [-3000 3000]);
end

if ishandle(p)
    %hold on
    set(p, 'XData', Pos1(1,:));
    set(p, 'YData', Pos1(2,:));
    %plot(Pos1(1,:), Pos1(2,:), 'ro', 'MarkerSize',5);
    %set(w, 'XData', Position(1));
    %set(w, 'YData', Position(2));
    drawnow limitrate;
end

== matlab function SIL_OlfatiSaber/Save Data/Formation Shape Plot ==
  data: Positions input; Positions_ant input; r_comm input; max_agent input
function plotFormation(Positions, Positions_ant, r_comm, max_agent)
coder.extrinsic('Formation_plot');
coder.extrinsic('compute_neighborhood');
persistent p;
%persistent w;

Pos1 = reshape(Positions,3,[]);
Pos2 = reshape(Positions_ant,3,[]);
M = compute_neighborhood(pdist(Pos1), r_comm, max_agent);

if isempty(p)
    %hold on
    p = figure;
    %p = plot(0, 0, 'ro', 'MarkerSize',15);
    %w = plot(Position(1), Position(2), 'b*');
    %hold off
    %set(gca,'XLim', [-3000 3000], 'YLim', [-3000 3000]);
end

if ishandle(p)
    Formation_plot(M, Pos2, Pos1, max_agent, p);
    %set(p, 'XData', WaypointX);
    %set(p, 'YData', WaypointY);
    %set(w, 'XData', Position(1));
    %set(w, 'YData', Position(2));
    drawnow limitrate;
end

== matlab function SIL_OlfatiSaber/UAV 4/High-level/Coordination Algorithm/Olfati-Saber Algorithm ==
  data: p_swarm_par input; pos input; vel input; u_ref input; dt input; r_agent input; vel_command output
function vel_command = compute_vel_olfati_saber(p_swarm_par, pos, vel, u_ref, dt, r_agent)
    
    %% swarm parameters
    % variables to be set
    p_swarm.is_active_migration = 1;
    p_swarm.is_active_arena = 0;
    p_swarm.is_active_spheres = 0;
    p_swarm.is_active_cyl = 0;
    
    % number of agents
    nb_agents = 5;
    
    % max radius of influence - metric distance
    p_swarm.r = p_swarm_par(2);
    
    % max number of neighbors - Topological distance
    p_swarm.max_neig = p_swarm_par(3);
    
    % radius of collision
    p_swarm.r_coll = p_swarm_par(4);
    
    % % Olfati-Saber parameters
    % coefficients for velocity matching
    p_swarm.c_vm = p_swarm_par(5);
    p_swarm.a = p_swarm_par(6);
    p_swarm.b = p_swarm_par(7);
    p_swarm.c = p_swarm_par(8); %(p_swarm.b-p_swarm.a)/(2*sqrt(p_swarm.a*p_swarm.b));
    p_swarm.delta = p_swarm_par(9);
    p_swarm.k = p_swarm_par(10);
    
    % obstacle parameters
    p_swarm.r0 = p_swarm_par(11);
    p_swarm.lambda = p_swarm_par(12); % (0,1]
    p_swarm.c_pm_obs = p_swarm_par(13);
    p_swarm.c_vm_obs = p_swarm_par(14); %p_swarm.c_vm;
    
    % wall parameters
    p_swarm.d_arena = p_swarm_par(15);
    p_swarm.c_arena = p_swarm_par(16);
    p_swarm.n_spheres = p_swarm_par(17);
    p_swarm.n_cyl = p_swarm_par(18);
    p_swarm.spheres = [-70 70 0; 50 50 200; 5 5 5; 50 50 50];
    p_swarm.x_arena = [-100   100; -100   100; -100   100];
    p_swarm.cylinders = [];
    
    % % Reference values

    % Inter-agent distance
    p_swarm.d_ref = p_swarm_par(19);
    
    % Velocity direction
    p_swarm.u_ref = u_ref;

    % Speed
    p_swarm.v_ref = p_swarm_par(20);
    
    % Velocity and acceleration bounds for the agents
    p_swarm.max_a = p_swarm_par(21);
    p_swarm.max_v = p_swarm_par(22);

    %% Initialize variables
    
    M = zeros(1, nb_agents);    % Neighborhood matrix
    D = zeros(1, nb_agents);    % Distance matrix
    acc_pm = zeros(3, 1);       % Position matching acceleration
    acc_vm = zeros(3, 1);       % Velocity matching acceleration
    acc_wall = zeros(3, 1);     % Arena repulsion acceleration
    acc_obs = zeros(3, 1);      % Obstacle repulsion acceleration
    acc_command = zeros(3, 1);  % Calculate the commanded acceleration
    vel_command = zeros(3, 1);  % Calculate the commanded velocity

    nb_agent_collisions = 0;    % Nb of collisions among agents
    nb_obs_collisions = 0;      % Nb of collisions against obstacles
    min_dist_obs = 20;          % Init minimum distance to obstacles

    %% Compute useful functions

    % Weight function for computing the motion planning acceleration
    psi = @(z) ((p_swarm.a + p_swarm.b) * (sqrt(1 + (z - p_swarm.d_ref + p_swarm.c)^2) - sqrt(1 + p_swarm.c^2)) + ...
        (p_swarm.a - p_swarm.b) * (z - p_swarm.d_ref)) / 2;
    psi_der = @(z) (p_swarm.a + p_swarm.b) / 2 * (z - p_swarm.d_ref + p_swarm.c) ./ sqrt(1 + (z - p_swarm.d_ref + p_swarm.c)^2) + ...
        (p_swarm.a - p_swarm.b) / 2;

    % Generalization of adjacency coefficients for computing the motion planning acceleration
    rho = @rho_f;
    rho_der = @rho_der_f;

    % Force defining the attraction/repulsion as function of the distance
    phi = @(z) 1 / p_swarm.r * rho_der(z, p_swarm.delta, p_swarm.r, p_swarm.k) * psi(z) + ...
        rho(z, p_swarm.delta, p_swarm.r, p_swarm.k) * psi_der(z);
   
%% Compute velocity commands for every agent
    
    for agent = 1:1
        
        
        %% Find neighbors
        
        % Compute agent-agent distance matrix
        % p_rel = pos - pos(:, agent);
        p_rel = zeros(3, nb_agents);
        for k = 1:nb_agents
            p_rel(:, k) = pos(:, k) - pos(:, agent);
        end
        
        dist = sqrt(sum((p_rel.^2), 1));
        D(agent, :) = dist;

        % Define neighbors list
        neig_lis = (1:nb_agents)';
        neig_lis = neig_lis(dist ~= 0);

        % Count collisions
        nb_agent_collisions = nb_agent_collisions + sum(dist < 2 * r_agent) - 1;

        % Number of neighbours
        nb_neig = nb_agents - 1;

        % Constraint on neighborhood given by the euclidean distance
        if isfield(p_swarm, 'r')
            neig_lis = neig_lis(dist(neig_lis) < p_swarm.r);
            nb_neig = length(neig_lis);
        end

        % Constraint on neighborhood given by the topological distance
        if isfield(p_swarm, 'max_neig')

            if nb_neig > p_swarm.max_neig
                [~, idx] = sort(dist(neig_lis));
                neig_lis = neig_lis(idx(1:p_swarm.max_neig));
                nb_neig = p_swarm.max_neig;
            end

        end

        % Adjacency matrix (asymmetric in case of limited fov)
        M(agent, neig_lis) = 1;

        
        %% Compute different contributions
        if nb_neig ~= 0
            % vel_rel = vel - vel(:, agent);
            vel_rel = zeros(3, nb_agents);
            for k = 1:nb_agents
                vel_rel(:, k) = vel(:, k) - vel(:, agent);
            end
            % v_rel_norm  = sqrt(sum((v_rel.^2),1));

            % Compute pos unit vector between two agents
            %pos_rel_u = p_rel ./ dist;
            pos_rel_u = zeros(3, nb_agents); 
            for k = 1:nb_agents
                if(k ~= agent)
                    pos_rel_u(:, k) = p_rel(:, k) ./ dist(k);
                end
            end
            
            for agent2 = 1:nb_agents
                % Position matching
                acc_pm(:, agent) = acc_pm(:, agent) + phi(dist(agent2)) * pos_rel_u(:, agent2);

                % Velocity matching
                if ~p_swarm.is_active_migration
                    acc_vm(:, agent) = acc_vm(:, agent) + p_swarm.c_vm * vel_rel(agent2);
                end
            end
        end

        % Add migration effect on accelerations
        if p_swarm.is_active_migration
            acc_vm(:, agent) = p_swarm.c_vm * (p_swarm.u_ref * p_swarm.v_ref - vel(:, agent));
        end
        
        
        %% Wall and obstacle avoidance

        % Add arena repulsion effect on accelerations
        if p_swarm.is_active_arena
            acc_wall(:, agent) = repulsion_cubic_arena(pos(:, agent), p_swarm.x_arena, p_swarm.d_arena, p_swarm.c_arena);
        end

        % Spheric obstacles effect
        if p_swarm.is_active_spheres

            for obs = 1:p_swarm.n_spheres
                % Get obstacle center and radius
                c_obs = p_swarm.spheres(1:3, obs);
                r_obs = p_swarm.spheres(4, obs);

                pos_agent = pos(:, agent);
                vel_agent = vel(:, agent);

                % Compute distance agent(a)-obstacle(b)
                dist_ab = sqrt(sum((pos(:, agent) - c_obs).^2)) - r_obs;
                nb_obs_collisions = nb_obs_collisions + sum(dist_ab < r_agent);

                if dist_ab < min_dist_obs
                    min_dist_obs = dist_ab;
                end

                if (dist_ab < p_swarm.r0)
                    % Parameter s in [0,1]
                    s = r_obs / (r_obs + dist_ab);
                    pos_obs = s * pos_agent + (1 - s) * c_obs;

                    % Derivative of s
                    s_dot = r_obs * (vel_agent' * (pos_obs - pos_agent) / dist_ab) / (r_obs + dist_ab)^2;
                    vel_obs = s * vel_agent - r_obs * (s_dot / s) * (pos_obs - pos_agent) / dist_ab;
                    pos_gamma = c_obs + p_swarm.lambda * p_swarm.u_ref;
                    d_ag = norm(pos_gamma - pos(:, agent));

                    % Acceleration effect
                    acc_obs(:, agent) = acc_obs(:, agent) + ...
                        +p_swarm.c_pm_obs * rho(dist_ab / p_swarm.r0, p_swarm.delta, p_swarm.r, p_swarm.k) * ...
                        (phi(dist_ab - p_swarm.d_ref) * (pos_obs - pos_agent) / dist_ab + ...
                        phi(d_ag - p_swarm.d_ref) * (pos_gamma - pos_agent) / (norm(pos_gamma - pos_agent))) + ...
                        p_swarm.c_vm_obs * (vel_obs - vel_agent);
                end
            end
        end

        % Cylindric obstacle effect
        if p_swarm.is_active_cyl

            for obs = 1:p_swarm.n_cyl
                % Get obstacle center and radius
                c_obs = p_swarm.cylinders(1:2, obs);
                r_obs = p_swarm.cylinders(3, obs);

                pos_agent = pos(1:2, agent);
                vel_agent = vel(1:2, agent);

                % Compute distance agent(a)-obstacle(b)
                dist_ab = sqrt(sum((pos(1:2, agent) - c_obs).^2)) - r_obs;
                nb_obs_collisions = nb_obs_collisions + sum(dist_ab < r_agent);

                if dist_ab < min_dist_obs
                    min_dist_obs = dist_ab;
                end

                % Compute interaction effect
                if (dist_ab < p_swarm.r0)
                    % Parameter s in [0,1]
                    s = r_obs / (r_obs + dist_ab);
                    pos_obs = s * pos_agent + (1 - s) * c_obs;

                    % Derivative of s
                    s_dot = r_obs * (vel_agent' * (pos_obs - pos_agent) / dist_ab) / (r_obs + dist_ab)^2;
                    vel_obs = s * vel_agent - r_obs * (s_dot / s) * (pos_obs - pos_agent) / dist_ab;
                    pos_gamma = c_obs + p_swarm.lambda * p_swarm.u_ref(1:2);
                    d_ag = norm(pos_gamma - pos(1:2, agent));

                    % Acceleration effect of the spheric obstacles
                    acc_obs(1:2, agent) = acc_obs(1:2, agent) + ...
                        +p_swarm.c_pm_obs * rho(dist_ab / p_swarm.r0, p_swarm.delta, p_swarm.r, p_swarm.k) * ...
                        (phi(dist_ab - p_swarm.d_ref) * (pos_obs - pos_agent) / dist_ab + ...
                        phi(d_ag - p_swarm.d_ref) * (pos_gamma - pos_agent) / (norm(pos_gamma - pos_agent))) + ...
                        p_swarm.c_vm_obs * (vel_obs - vel_agent);
                end

            end

        end
        
        %% Sum contributions
        acc_command(:, agent) = acc_pm(:, agent) + acc_vm(:, agent) + acc_wall(:, agent) + acc_obs(:, agent); 
        
        % Integrate acceleration to get velocity
        vel_command(:, agent) = vel(:, agent) + acc_command(:, agent) * dt;
        
    end
    
    %% Compute collisions and bound velocities and accelerations
    
    % Add random effect on velocities
    if isfield(p_swarm, 'c_r')
        vel_command = vel_command + p_swarm.c_r * randn(3, nb_agents);
    end

    % Bound velocities
    if isempty(p_swarm.max_v)
        v_norm = sqrt(sum((vel_command.^2), 1));
        idx_to_bound = (v_norm > p_swarm.max_v);

        if sum(idx_to_bound) > 0
            vel_command(:, idx_to_bound) = p_swarm.max_v * ...
                vel_command(:, idx_to_bound) ./ repmat(v_norm(idx_to_bound), 3, 1);
        end
    end
    if isempty(p_swarm.max_a)
        accel_cmd = (vel_command-vel)./dt;
        accel_cmd_norm = sqrt(sum(accel_cmd.^2, 1));
        idx_to_bound = ( accel_cmd_norm > p_swarm.max_a | accel_cmd_norm < - p_swarm.max_a);
        if sum(idx_to_bound) > 0
            vel_command(:, idx_to_bound) = vel(:, idx_to_bound) + ...
                dt*p_swarm.max_a * accel_cmd(:, idx_to_bound) ./ ...
                repmat(accel_cmd_norm(idx_to_bound), 3, 1);
        end
    end

end

%%%%%%%%%%%%%%%%%%%%%%%%%%%%%%%%%%%%%%%%%%%%%%%%%%
% RHO - It is the function defining the adjacency coefficients
%
%%%%%%%%%%%%%%%%%%%%%%%%%%%%%%%%%%%%%%%%%%%%%%%%%%

function y = rho_f(z, delta, r, k)

    if z < delta * r
        y = 1;
        return;
    elseif z < r
        y = (1/2^k) * (1 + cos(pi * (z / r - delta) ./ (1 - delta)))^k;
        return;
    else
        y = 0;
    end

end

%%%%%%%%%%%%%%%%%%%%%%%%%%%%%%%%%%%%%%%%%%%%%%%%%%
% Derivative of rho
%
%%%%%%%%%%%%%%%%%%%%%%%%%%%%%%%%%%%%%%%%%%%%%%%%%%

function y = rho_der_f(z, delta, r, k)

    if z < delta * r
        y = 0;
        return;
    elseif z < r
        arg = pi * (z / r - delta) ./ (1 - delta);
        y = -pi / (1 - delta) * k / (2^k) * (1 + cos(arg))^(k - 1) * (sin(arg));
        return;
    else
        y = 0;
    end

end

%%%%%%%%%%%%%%%%%%%%%%%%%%%%%%%%%%%%%%%%%%%%%%%%%%
% Repulsion from cubic arena
%
%%%%%%%%%%%%%%%%%%%%%%%%%%%%%%%%%%%%%%%%%%%%%%%%%%

function a_arena = repulsion_cubic_arena(pos_drone, pos_walls, wall_width, const_rep)

    a_arena = zeros(3, 1);

    for axis = 1:3
        x_drone = pos_drone(axis);
        % Repulsion from left wall
        x_arena = pos_walls(axis, 1);

        if x_drone < x_arena
            a_arena(axis) = a_arena(axis) + const_rep;
        elseif x_drone > x_arena && x_drone < x_arena + wall_width
            a_arena(axis) = a_arena(axis) + const_rep * 0.5 * (sin((pi / wall_width) * (x_drone + x_arena) + pi / 2) + 1);
        end

        % Repulsion from right wall
        x_arena = pos_walls(axis, 2);

        if x_drone > x_arena - wall_width && x_drone < x_arena
            a_arena(axis) = a_arena(axis) - const_rep * 0.5 * (sin((pi / wall_width) * (x_drone - x_arena - wall_width) - pi / 2) + 1);
        elseif x_drone > x_arena
            a_arena(axis) = a_arena(axis) - const_rep;
        end

    end

end

== matlab function SIL_OlfatiSaber/UAV 4/High-level/Network/Status Network ==
  data: N_Agents input; Wifi_Scan input; SignalDbms output
% this function is a union of data of uav i and your neighbors
function SignalDbms = Wifi_Signal(N_Agents, Wifi_Scan)
    SignalDbms = zeros(1, 5);
    Ssids = zeros(1, 5);
    Frequencys = zeros(1, 5);
    
    for i=1:N_Agents
        SignalDbms(i) = Wifi_Scan.Signals(i).SignalDbm;
        %Ssids(i) = Wifi_Scan.Signals(i).Ssid;
        %Frequencys(i) = Wifi_Scan.Signals(i).Frequency;
    end
end

== matlab function SIL_OlfatiSaber/UAV 4/High-level/Waypoint Generator/Velocity Direction ==
  data: pos input; wp input; u_ref output
function u_ref = velocity_direction(pos, wp)
    pos_mean_rel = wp - pos;
    
    r = sqrt( sum( pos_mean_rel.^2 ) );
    x = pos_mean_rel(1);
    y = pos_mean_rel(2);
    %z = pos_mean_rel(3)/r;
    
    orientation = atan2(y,x);
    u_ref = [cos(orientation); sin(orientation); 0];

end

== matlab function SIL_OlfatiSaber/UAV 4/High-level/Waypoint Generator/Waypoint Algorithm ==
  data: Xi input; R input; p_swarm_r input; Waypoints input; N_Waypoints input; wp output; Current_Waypoint output; Current_Waypoint input
function [wp, Current_Waypoint] = Next_Waypoint(Xi, R, p_swarm_r, Waypoints, N_Waypoints, Current_Waypoint)

    X_ref = Waypoints(Current_Waypoint + 1, 1);
    Y_ref = Waypoints(Current_Waypoint + 1, 2);
    wp = [X_ref; Y_ref; 0];

    if ( is_visited(Xi, R, p_swarm_r, X_ref, Y_ref)  )
        Current_Waypoint = mod(Current_Waypoint + 1, N_Waypoints);
    else
        Current_Waypoint = mod(Current_Waypoint, N_Waypoints);
    end

end

function visited = is_visited(Xi, R, p_swarm_r, wp1_X,wp1_Y)
    visited = 0;
    N = size(Xi,2);
    
    for i=1:N
        % if the aircraft inter the communication range and acces the
        % waypoitn area
        if( sqrt( (Xi(1, 1) - Xi(1, i) )^2 +(Xi(2, 1) - Xi(2, i))^2) < p_swarm_r && sqrt( (wp1_X - Xi(1, i) )^2 +(wp1_Y - Xi(2, i))^2) < R )
            visited = 1;
            return
        end
    end
    
end

== matlab function SIL_OlfatiSaber/UAV 4/Low-level/ROS Settings/Wi-Fi frame to Matrix ==
  data: nb_agents input; pos_i input; pos output; pqj input
% this function is a union of data of uav i and your neighbors
function pos = uavs_data(nb_agents, pos_i, pqj)
    %% Create Matrix pj and qj neighbors
    nb_agents = 5;
    
    pos = zeros(3, nb_agents);  % 
    %vel = zeros(3, nb_agents);  % 
    
    % position of agent i
    pos(:,1) = pos_i; % Posição
    %vel(:,1) = vel_i; % Velocidade
    
    % neighbors of i
    for j=1:nb_agents-1
         %id_j = pqj(j).Id;
         pos(:,j+1) = [pqj(j).X; pqj(j).Y; pqj(j).Z]; % Posição
         %vel(:,j+1) = [pqj(j).VelocityX; pqj(j).VelocityY; pqj(j).VelocityZ]; % Velocidade
    end

end
